simulink model "SimTrifasicoMeioLinhaMonofasico"  (R2022b)
settings: Solver=ode45  StartTime=0.0  StopTime=SimulacaoTempo  RelTol=1e-3  EnableMultiTasking=on
values from neighbouring files (symbols this model uses):
  C_matrix = [7.14789431755e-09  -2.14393248907e-09; -2.14393248907e-09  7.14789431755e-09]    [Modelo2fios2awg160.mat]    (also in trifasico2awg.mat = [7.86602198725e-09  -2.45195546694e-09  -1.42580481937e-09; ; trifasico2awgNew.mat = [8.93900996847e-09  -2.36457299077e-09  -1.26282974561e-09; )
  dd = [ 20 ]    [CarregaDados20km.m]
  L_matrix = [0.00251001340283  0.00125944754059; 0.00125944754059  0.00251001340283]    [Modelo2fios2awg160.mat]    (also in trifasico2awg.mat = [0.00242085814129  0.00130892171515  0.00117029227904; 0.001; trifasico2awgNew.mat = [0.0018119254645  0.000784575768319  0.000670213848675; 0.00)
  m1 = n    [CurtoCircuitos.m]    (also in CurtosComparadosMonofasicos.m)
  R_matrix = [1.15977689742  0.0576982604784; 0.0576982604784  1.15977689742]    [Modelo2fios2awg160.mat]    (also in trifasico2awg.mat = [1.15895092862  0.0568724513894  0.0568719145431; 0.05687245; trifasico2awgNew.mat = [0.213716566428  0.0989824596492  0.099050906555; 0.09898245)
  TrifTerra = ValorCurto    [CurtosComparadosMonofasicos.m]
  TrifTestA = 1e6    (= 1000000)    [CurtosComparadosMonofasicos.m]
  TrifTestB = 1e-5    (= 1e-05)    [CurtosComparadosMonofasicos.m]
  TrifTestC = 1e6    (= 1000000)    [CurtosComparadosMonofasicos.m]
undefined symbols (not defined in the file or in its folder): D11, Delta
libraries: spsSeriesRLCBranchLib x4, spsDistributedParametersLineLib x2, spsGroundLib x1, spsThreePhaseVIMeasurementLib x1, spsThreePhaseTransformerTwoWindingsLib x1, spsThreePhaseSourceLib x1, spspowerguiLib x1
settings Model: Creator=laris  LastModifiedBy=Leonardo-Felipe
settings SolverCC: AlgebraicLoopSolver=TrustRegion
settings DataIOCC: LimitDataPoints=on  SaveFormat=Array  ReturnWorkspaceOutputs=off
settings OptimizationCC: LifeSpan=inf
settings DebuggingCC: UnconnectedInputMsg=warning  UnconnectedOutputMsg=warning  UnconnectedLineMsg=warning  SFUnexpectedBacktrackingDiag=warning  SFNoUnconditionalDefaultTransitionDiag=warning  SFExecutionAtInitializationDiag=none  SFMachineParentedDataDiag=warning  ArithmeticOperatorsInVariantConditions=warning
settings HardwareCC: ProdBitPerPointer=32  ProdBitPerSizeT=32  ProdBitPerPtrDiffT=32  ProdLargestAtomicFloat=None  ProdIntDivRoundTo=Undefined  ProdEndianess=Unspecified  ProdWordSize=32  ProdHWDeviceType=32-bit Generic
settings ModelReferenceCC: EnableRefExpFcnMdlSchedulingChecks=on  PropagateSignalLabelsOutOfModel=off
settings SFSimCC: SimUseLocalCustomCode=off  CustomCodeUndefinedFunction=UseInterfaceOnly
settings RTWCC: RTWUseLocalCustomCode=off  DLArmComputeVersion=19.05
settings CodeAppCC: StateflowObjectComments=on
settings GRTTargetCC: TargetLangStandard=C89/C90 (ANSI)
settings ConfigComp: CovMetricSettings=dw  CovSaveCumulativeToWorkspaceVar=on  CovSaveSingleToWorkspaceVar=on  CovExternalEMLEnable=off
settings SimscapeCC: SimscapeNormalizeSystem=off

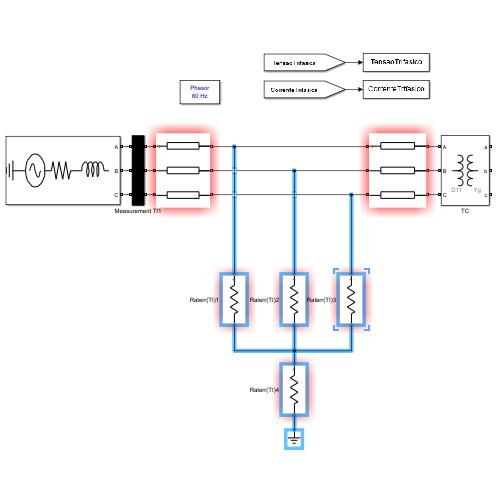
[thumbnail: Simulink's stored preview of the top-level diagram]
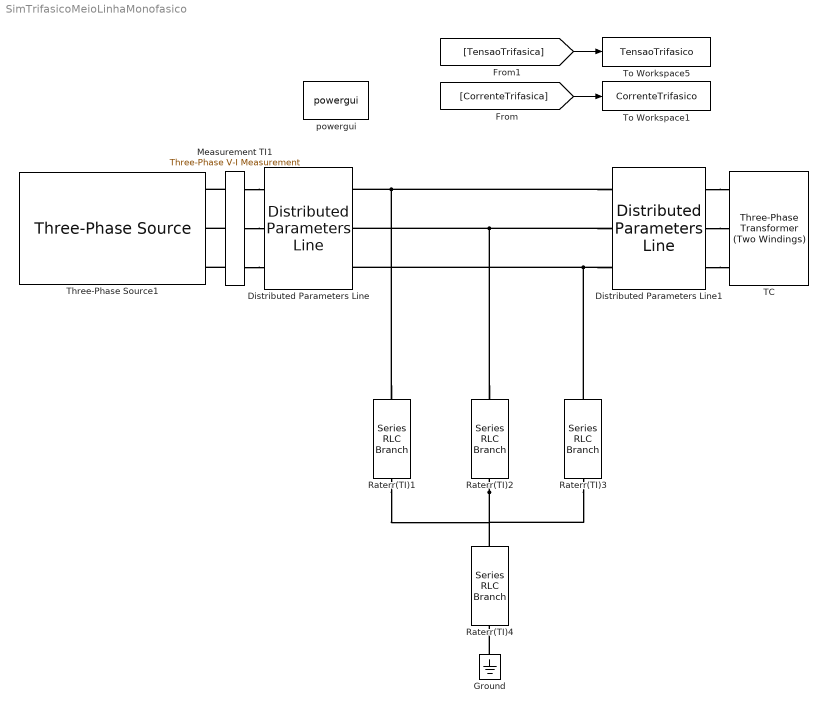
== system SimTrifasicoMeioLinhaMonofasico ==
  Distributed Parameters Line : spsDistributedParametersLineLib/Distributed Parameters Line  Phases=3  Length=dd * m1  Frequency=60  Resistance=R_matrix  Inductance=L_matrix  Capacitance=C_matrix  x1=[432.778243523007 7105.70811875224 14056.356481723;376.991118430775 376.991118430775 376.991118430775;-2.09542283136629 -1.42726330950845 -2.09745137758092]  x2=[432.7786479799 7104.77267952713 14056.3645449837;376.991118430775 376.991118430775 376.991118430775;-2.09542351119504 -1.42732127431346 -2.0974530293211]  x3=[0.381725288016439 122.744172782181 45.2664542751573;376.991118430775 376.991118430775 376.991118430775;-2.19261875491375 1.72646893240697 -2.17467656928648]  x4=[0.383944871738965 161.47668910103 45.3724490059456;376.991118430775 376.991118430775 376.991118430775;-1.99880102268865 -1.41804354940171 -2.0204163368923]  x5=2.60355177502627e-08  V1=ones(3,3)  V2=ones(3,3)  I1=ones(3,3)  I2=ones(3,3)  nHarmo=1  Measurements=None  Decoupling=on  VsMag0=[3607.07330409513 11480.9278370979 10173.5494845166]  VrMag0=[3606.69950937585 11480.934516926 10173.0323046331]  VsAngle0=[-0.0972552378502089 -120.172016309447 77.686730664022]  VrAngle0=[-0.0875607854643758 -120.172109677148 77.6838301447826]  IsMag0=[101.501548376663 36.3199225857195 74.1174140752129]  IrMag0=[99.0074935270974 36.4057489355303 130.405612827982]  IsAngle0=[91.4766511296065 -124.605842881636 -70.8615332676647]  IrAngle0=[-74.9557376532867 -115.753029093636 93.9797543202312]
  Distributed Parameters Line1 : spsDistributedParametersLineLib/Distributed Parameters Line  Phases=3  Length=dd * (1-m1)  Frequency=60  Resistance=R_matrix  Inductance=L_matrix  Capacitance=C_matrix  x1=[432.7786479799 7104.77267952713 14056.3645449837;376.991118430775 376.991118430775 376.991118430775;-2.19355547043309 -1.50441150393532 -2.17489780020318]  x2=[434.792989999328 7125.14792818239 14097.0039950559;376.991118430775 376.991118430775 376.991118430775;-2.19691844061339 -1.5113535110284 -2.18312055868034]  x3=[0.363636227669757 16.9740236366004 38.6713570856884;376.991118430775 376.991118430775 376.991118430775;-2.2925553008553 -1.58474016683204 -2.25626269876542]  x4=[0.364589028883781 16.9890880202982 38.7018861186386;376.991118430775 376.991118430775 376.991118430775;-2.19783669338111 -1.51164065074527 -2.18336600080964]  x5=0.000260329141984877  V1=ones(3,3)  V2=ones(3,3)  I1=ones(3,3)  I2=ones(3,3)  nHarmo=1  Measurements=None  Decoupling=on  VsMag0=[3606.69950937585 11480.934516926 10173.0323046331]  VrMag0=[3624.31464970068 11514.5837338414 10199.2966229041]  VsAngle0=[-0.0875607854643758 -120.172109677148 77.6838301447826]  VrAngle0=[-0.557339102245022 -120.636877798051 77.2407535013352]  IsMag0=[11.3294706246617 34.5180745629362 29.5772252753248]  IrMag0=[11.3439999175504 34.5457618619082 29.5990763493586]  IsAngle0=[9.04923899095949 -124.842485106729 71.2025147788419]  IrAngle0=[13.2004691770678 -120.657615944921 75.376519113798]
  Ground : spsGroundLib/Ground  LConnTagsString=a
  Measurement TI1 : spsThreePhaseVIMeasurementLib/Three-Phase V-I Measurement  VoltageMeasurement=phase-to-phase  SetLabelV=on  LabelV=TensaoTrifasica  Vpu=off  VpuLL=off  CurrentMeasurement=yes  SetLabelI=on  LabelI=CorrenteTrifasica  Ipu=off  Pbase=100e6  Vbase=500e3  OutputType=Complex  PhasorSimulation=on  PSBequivalent=0
  Raterr(TI)1 : spsSeriesRLCBranchLib/Series RLC Branch  LConnTagsString=__new0  RConnTagsString=__new0  BranchType=R  Resistance=TrifTestA  Inductance=0  SetiL0=off  InitialCurrent=0  Capacitance=1e-6  Setx0=off  InitialVoltage=0  Measurements=None
  Raterr(TI)2 : spsSeriesRLCBranchLib/Series RLC Branch  LConnTagsString=__new0  RConnTagsString=__new0  BranchType=R  Resistance=TrifTestB  Inductance=0  SetiL0=off  InitialCurrent=0  Capacitance=1e-6  Setx0=off  InitialVoltage=0  Measurements=None
  Raterr(TI)3 : spsSeriesRLCBranchLib/Series RLC Branch  LConnTagsString=__new0  RConnTagsString=__new0  BranchType=R  Resistance=TrifTestC  Inductance=0  SetiL0=off  InitialCurrent=0  Capacitance=1e-6  Setx0=off  InitialVoltage=0  Measurements=None
  Raterr(TI)4 : spsSeriesRLCBranchLib/Series RLC Branch  LConnTagsString=__new0  RConnTagsString=__new0  BranchType=R  Resistance=TrifTerra  Inductance=0  SetiL0=off  InitialCurrent=0  Capacitance=1e-6  Setx0=off  InitialVoltage=0  Measurements=None
  TC : spsThreePhaseTransformerTwoWindingsLib/Three-Phase Transformer (Two Windings)  Winding1Connection=Delta (D11)  Winding2Connection=Yg  CoreType=Three single-phase transformers  SetSaturation=off  Hysteresis=off  DataFile='hysteresis'  SetInitialFlux=off  Measurements=None  UNITS=pu  NominalPower=[120e3 , 60]  Winding1=[13800 0.0048118 0.018511]  Winding2=[380 0.0048119 0.018511]  Rm=5.801193266567229e+02  Lm=8.409977380031759e+02  L0=0.50001  Saturation=[0 0;0.0012545 0.01913;0.52272 0.024231]  InitialFluxes=[0.66025 -0.66025 0.57768]  BreakLoop=off  DiscreteSolver=Trapezoidal iterative  DataType=off  TransfoNumber=1
  Three-Phase Source1 : spsThreePhaseSourceLib/Three-Phase Source  InternalConnection=Yg  VoltagePhases=off  Voltage=13.8e3  PhaseAngle=0  Voltage_phases=[25e3 25e3 25e3]/sqrt(3)  PhaseAngles_phases=[0 -120 +120]  Frequency=60  NonIdealSource=on  SpecifyImpedance=on  Resistance=0.8929  Inductance=16.58e-3  ShortCircuitLevel=2.5e6  BaseVoltage=13.8e3  XRratio=7  BusType=swing  Pref=10e3  Qref=0  Prefabc=[10e3, 10e3, 10e3]  Qrefabc=[0, 0, 0]  Qmin=-inf  Qmax=inf
  To Workspace1 : ToWorkspace  VariableName=CorrenteTrifasico  SampleTime=-1
      settings: MaxDataPoints=1
  To Workspace5 : ToWorkspace  VariableName=TensaoTrifasico  SampleTime=-1
      settings: MaxDataPoints=1
  powergui : spspowerguiLib/powergui  Priority=1  SimulationMode=Phasor  SampleTime=50e-9  frequency=60  Iterations=50  frequencyindice=60  Pbase=100e6  ErrMax=1e-4  UnitsV=kV  UnitsW=MW  buscounter=0  FunctionMessages=off  echomessages=off  EnableUseOfTLC=off  CurrentSourceSwitches=off  DisableSnubberDevices=off  DisableRonSwitches=off  DisableVfSwitches=off  DisplayEquations=off  AutomaticDiscreteSolvers=off  SolverType=Tustin/Backward Euler (TBE)  Interpol=off  ExternalGateDelay=off  methode=off  Ts=100  x0status=blocks  SPID=on  SwTol=0  HookPort=off  NonlinearTolerance=1e-4  nMaxIteration=100  ContinueOnMaxIteration=off  RestoreLinks=warning  ResistiveCurrentMeasurement=off  Frange=[0:2:500]  Ylog=off  Xlog=on  ShowGrid=off  save=off  variable=ZData  structure=0  ZoomFFT=off  StartTime=0.0  cycles=1  DisplayStyle=1  fundamental=60  FreqAxis=off  MaxFrequency=1000  frequencyindicesteady=1  RmsSteady=1  display=off
  wires:
  [TensaoTrifasica] -> To Workspace5/1
  [CorrenteTrifasica] -> To Workspace1/1
  connections:
  Distributed Parameters Line1/LConn2 -- Raterr(TI)2/LConn1 -- Distributed Parameters Line/RConn2
  Distributed Parameters Line1/RConn1 -- TC/LConn1
  Distributed Parameters Line1/RConn2 -- TC/LConn2
  Distributed Parameters Line1/RConn3 -- TC/LConn3
  Distributed Parameters Line1/LConn3 -- Raterr(TI)3/LConn1 -- Distributed Parameters Line/RConn3
  Distributed Parameters Line1/LConn1 -- Distributed Parameters Line/RConn1 -- Raterr(TI)1/LConn1
  Raterr(TI)2/RConn1 -- Raterr(TI)4/LConn1 -- Raterr(TI)1/RConn1 -- Raterr(TI)3/RConn1
  Measurement TI1/LConn1 -- Three-Phase Source1/RConn1
  Measurement TI1/LConn3 -- Three-Phase Source1/RConn3
  Measurement TI1/LConn2 -- Three-Phase Source1/RConn2
  Measurement TI1/RConn2 -- Distributed Parameters Line/LConn2
  Measurement TI1/RConn1 -- Distributed Parameters Line/LConn1
  Measurement TI1/RConn3 -- Distributed Parameters Line/LConn3
  Ground/LConn1 -- Raterr(TI)4/RConn1
